simulink model "v09_threebit_mult"  (R2019b)
settings: Solver=FixedStepAuto  StartTime=0.0  StopTime=inf  FixedStep=1  MaxStep=1  RelTol=1e-3
libraries: simulink x6
settings Model: Creator=MARAT  LastModifiedBy=Marat
settings SFSimCC: CustomCodeUndefinedFunction=UseInterfaceOnly

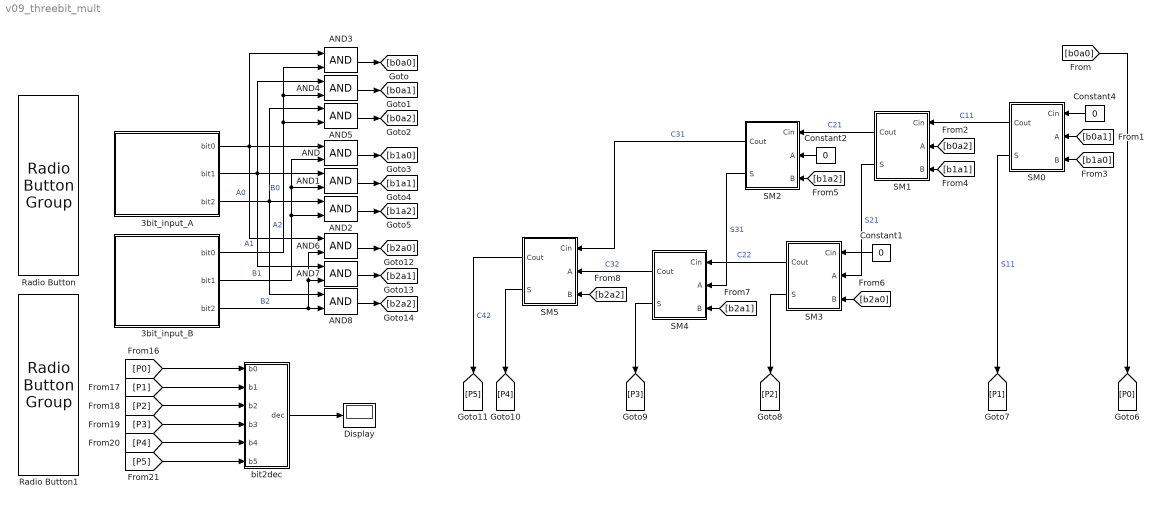
== system v09_threebit_mult ==
  3bit_input_A : Subsystem
      mask Display: image('images\sansA.png'); % Use "Edit Image" on toolstrip to change.
  3bit_input_B : Subsystem
      mask Display: image('images\sansB.png'); % Use "Edit Image" on toolstrip to change.
  AND{,1..8} (9 alike) : Logic  AllPortsSameDT=off  OutDataTypeStr=boolean
  Constant1 : Constant  Value=0  OutDataTypeStr=boolean
  Constant2 : Constant  Value=0  OutDataTypeStr=boolean
  Constant4 : Constant  Value=0  OutDataTypeStr=boolean
  Display : Display
  Radio Button : RadioButtonGroup  SelectedLabel=0
      settings: Values={{'0', '1', '2', '3', '4', '5', '6', '7'}, [0 1 2 3 4 5 6 7]}
  Radio Button1 : RadioButtonGroup  SelectedLabel=0
      settings: Values={{'0', '1', '2', '3', '4', '5', '6', '7'}, [0 1 2 3 4 5 6 7]}
  SM0 : Subsystem
  SM1 : Subsystem
  SM2 : Subsystem
  SM3 : Subsystem
  SM4 : Subsystem
  SM5 : Subsystem
  bit2dec : Subsystem
  wires:
  Constant4/1 -> SM0/1(Cin)
  [b0a0] -> [P0]
  3bit_input_A/1(bit0) -> AND6/1, AND/1, AND3/1  "A0"
  3bit_input_A/3(bit2) -> AND8/1, AND5/1, AND2/1  "A2"
  3bit_input_B/2(bit1) -> AND2/2, AND1/2, AND/2  "B1"
  [P0] -> bit2dec/1(b0)
  [P1] -> bit2dec/2(b1)
  [P2] -> bit2dec/3(b2)
  [P3] -> bit2dec/4(b3)
  [P4] -> bit2dec/5(b4)
  [P5] -> bit2dec/6(b5)
  bit2dec/1(dec) -> Display/1
  3bit_input_B/3(bit2) -> AND6/2, AND7/2, AND8/2  "B2"
  SM0/2(S) -> [P1]  "S11"
  SM1/1(Cout) -> SM2/1(Cin)  "C21"
  SM1/2(S) -> SM3/2(A)  "S21"
  SM3/2(S) -> [P2]
  SM3/1(Cout) -> SM4/1(Cin)  "C22"
  SM2/2(S) -> SM4/2(A)  "S31"
  SM4/2(S) -> [P3]
  3bit_input_A/2(bit1) -> AND7/1, AND4/1, AND1/1  "A1"
  3bit_input_B/1(bit0) -> AND3/2, AND4/2, AND5/2  "B0"
  AND3/1 -> [b0a0]
  AND4/1 -> [b0a1]
  AND5/1 -> [b0a2]
  AND2/1 -> [b1a2]
  AND1/1 -> [b1a1]
  AND/1 -> [b1a0]
  AND6/1 -> [b2a0]
  AND7/1 -> [b2a1]
  AND8/1 -> [b2a2]
  [b1a0] -> SM0/3(B)
  [b0a1] -> SM0/2(A)
  [b1a1] -> SM1/3(B)
  [b0a2] -> SM1/2(A)
  [b1a2] -> SM2/3(B)
  [b2a1] -> SM4/3(B)
  [b2a0] -> SM3/3(B)
  SM0/1(Cout) -> SM1/1(Cin)  "C11"
  Constant2/1 -> SM2/2(A)
  SM2/1(Cout) -> SM5/1(Cin)  "C31"
  [b2a2] -> SM5/3(B)
  SM4/1(Cout) -> SM5/2(A)  "C32"
  SM5/2(S) -> [P4]
  SM5/1(Cout) -> [P5]  "C42"
  Constant1/1 -> SM3/1(Cin)

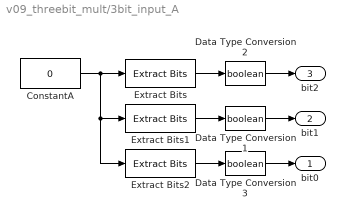
== system v09_threebit_mult/3bit_input_A ==
  ConstantA : Constant  Value=0  OutMin=0  OutMax=7  OutDataTypeStr=uint8
  Data Type Conversion1 : DataTypeConversion  OutDataTypeStr=boolean
  Data Type Conversion2 : DataTypeConversion  OutDataTypeStr=boolean
  Data Type Conversion3 : DataTypeConversion  OutDataTypeStr=boolean
  Extract Bits : simulink/Logic and Bit Operations/Extract Bits  bitsToExtract=Range of bits  numBits=8  bitIdxRange=2  outScalingMode=Treat bit field as an integer
      settings: SourceProductName=Simulink
  Extract Bits1 : simulink/Logic and Bit Operations/Extract Bits  bitsToExtract=Range of bits  numBits=8  bitIdxRange=1  outScalingMode=Treat bit field as an integer
      settings: SourceProductName=Simulink
  Extract Bits2 : simulink/Logic and Bit Operations/Extract Bits  bitsToExtract=Range of bits  numBits=8  bitIdxRange=0  outScalingMode=Treat bit field as an integer
      settings: SourceProductName=Simulink
  bit0 : Outport
  bit1 : Outport  Port=2
  bit2 : Outport  Port=3
  wires:
  ConstantA/1 -> Extract Bits2/1, Extract Bits1/1, Extract Bits/1
  Extract Bits/1 -> Data Type Conversion2/1
  Extract Bits1/1 -> Data Type Conversion1/1
  Extract Bits2/1 -> Data Type Conversion3/1
  Data Type Conversion2/1 -> bit2/1
  Data Type Conversion1/1 -> bit1/1
  Data Type Conversion3/1 -> bit0/1

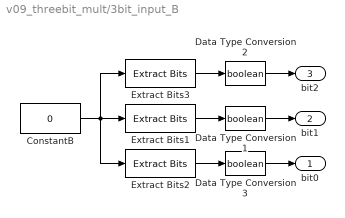
== system v09_threebit_mult/3bit_input_B ==
  ConstantB : Constant  Value=0  OutMin=0  OutMax=7  OutDataTypeStr=uint8
  Data Type Conversion1 : DataTypeConversion  OutDataTypeStr=boolean
  Data Type Conversion2 : DataTypeConversion  OutDataTypeStr=boolean
  Data Type Conversion3 : DataTypeConversion  OutDataTypeStr=boolean
  Extract Bits1 : simulink/Logic and Bit Operations/Extract Bits  bitsToExtract=Range of bits  numBits=8  bitIdxRange=1  outScalingMode=Treat bit field as an integer
      settings: SourceProductName=Simulink
  Extract Bits2 : simulink/Logic and Bit Operations/Extract Bits  bitsToExtract=Range of bits  numBits=8  bitIdxRange=0  outScalingMode=Treat bit field as an integer
      settings: SourceProductName=Simulink
  Extract Bits3 : simulink/Logic and Bit Operations/Extract Bits  bitsToExtract=Range of bits  numBits=8  bitIdxRange=2  outScalingMode=Treat bit field as an integer
      settings: SourceProductName=Simulink
  bit0 : Outport
  bit1 : Outport  Port=2
  bit2 : Outport  Port=3
  wires:
  Data Type Conversion3/1 -> bit0/1
  Data Type Conversion1/1 -> bit1/1
  Extract Bits2/1 -> Data Type Conversion3/1
  Extract Bits1/1 -> Data Type Conversion1/1
  ConstantB/1 -> Extract Bits3/1, Extract Bits1/1, Extract Bits2/1
  Extract Bits3/1 -> Data Type Conversion2/1
  Data Type Conversion2/1 -> bit2/1

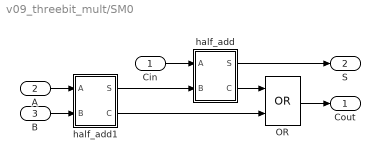
== system v09_threebit_mult/SM0 ==
  Cin : Inport
  A : Inport  Port=2
  B : Inport  Port=3
  OR : Logic  Operator=OR  AllPortsSameDT=off  OutDataTypeStr=boolean
  half_add : Subsystem
  half_add1 : Subsystem
  Cout : Outport
  S : Outport  Port=2
  wires:
  half_add/1(S) -> S/1
  A/1 -> half_add1/1(A)
  half_add/2(C) -> OR/1
  half_add1/1(S) -> half_add/2(B)
  B/1 -> half_add1/2(B)
  Cin/1 -> half_add/1(A)
  OR/1 -> Cout/1
  half_add1/2(C) -> OR/2

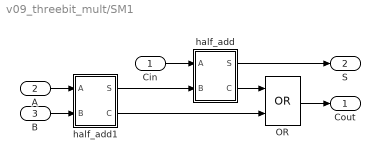
== system v09_threebit_mult/SM1 ==
  Cin : Inport
  A : Inport  Port=2
  B : Inport  Port=3
  OR : Logic  Operator=OR  AllPortsSameDT=off  OutDataTypeStr=boolean
  half_add : Subsystem
  half_add1 : Subsystem
  Cout : Outport
  S : Outport  Port=2
  wires:
  half_add1/2(C) -> OR/2
  OR/1 -> Cout/1
  Cin/1 -> half_add/1(A)
  B/1 -> half_add1/2(B)
  half_add1/1(S) -> half_add/2(B)
  half_add/2(C) -> OR/1
  A/1 -> half_add1/1(A)
  half_add/1(S) -> S/1

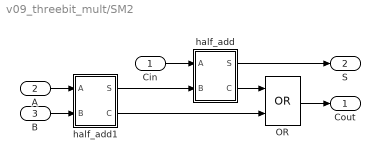
== system v09_threebit_mult/SM2 ==
  Cin : Inport
  A : Inport  Port=2
  B : Inport  Port=3
  OR : Logic  Operator=OR  AllPortsSameDT=off  OutDataTypeStr=boolean
  half_add : Subsystem
  half_add1 : Subsystem
  Cout : Outport
  S : Outport  Port=2
  wires:
  half_add/1(S) -> S/1
  A/1 -> half_add1/1(A)
  half_add/2(C) -> OR/1
  half_add1/1(S) -> half_add/2(B)
  B/1 -> half_add1/2(B)
  Cin/1 -> half_add/1(A)
  OR/1 -> Cout/1
  half_add1/2(C) -> OR/2

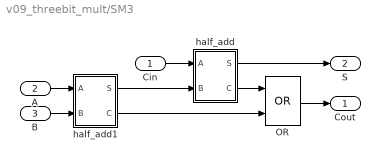
== system v09_threebit_mult/SM3 ==
  Cin : Inport
  A : Inport  Port=2
  B : Inport  Port=3
  OR : Logic  Operator=OR  AllPortsSameDT=off  OutDataTypeStr=boolean
  half_add : Subsystem
  half_add1 : Subsystem
  Cout : Outport
  S : Outport  Port=2
  wires:
  half_add1/2(C) -> OR/2
  OR/1 -> Cout/1
  Cin/1 -> half_add/1(A)
  B/1 -> half_add1/2(B)
  half_add1/1(S) -> half_add/2(B)
  half_add/2(C) -> OR/1
  A/1 -> half_add1/1(A)
  half_add/1(S) -> S/1

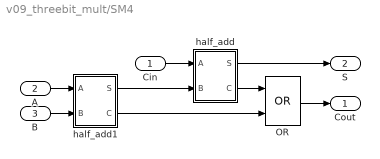
== system v09_threebit_mult/SM4 ==
  Cin : Inport
  A : Inport  Port=2
  B : Inport  Port=3
  OR : Logic  Operator=OR  AllPortsSameDT=off  OutDataTypeStr=boolean
  half_add : Subsystem
  half_add1 : Subsystem
  Cout : Outport
  S : Outport  Port=2
  wires:
  half_add/1(S) -> S/1
  A/1 -> half_add1/1(A)
  half_add/2(C) -> OR/1
  half_add1/1(S) -> half_add/2(B)
  B/1 -> half_add1/2(B)
  Cin/1 -> half_add/1(A)
  OR/1 -> Cout/1
  half_add1/2(C) -> OR/2

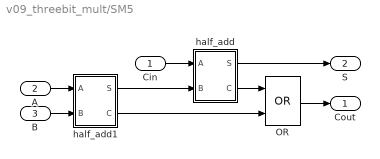
== system v09_threebit_mult/SM5 ==
  Cin : Inport
  A : Inport  Port=2
  B : Inport  Port=3
  OR : Logic  Operator=OR  AllPortsSameDT=off  OutDataTypeStr=boolean
  half_add : Subsystem
  half_add1 : Subsystem
  Cout : Outport
  S : Outport  Port=2
  wires:
  half_add1/2(C) -> OR/2
  OR/1 -> Cout/1
  Cin/1 -> half_add/1(A)
  B/1 -> half_add1/2(B)
  half_add1/1(S) -> half_add/2(B)
  half_add/2(C) -> OR/1
  A/1 -> half_add1/1(A)
  half_add/1(S) -> S/1

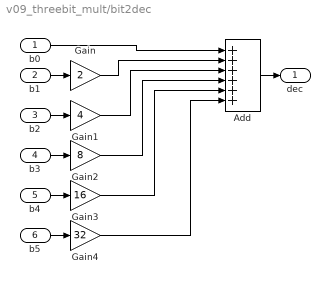
== system v09_threebit_mult/bit2dec ==
  b0 : Inport
  b1 : Inport  Port=2
  b2 : Inport  Port=3
  b3 : Inport  Port=4
  b4 : Inport  Port=5
  b5 : Inport  Port=6
  Add : Sum  Inputs=++++++
  Gain : Gain  Gain=2
  Gain1 : Gain  Gain=4
  Gain2 : Gain  Gain=8
  Gain3 : Gain  Gain=16
  Gain4 : Gain  Gain=32
  dec : Outport
  wires:
  b1/1 -> Gain/1
  b3/1 -> Gain2/1
  b2/1 -> Gain1/1
  b0/1 -> Add/1
  Add/1 -> dec/1
  Gain/1 -> Add/2
  Gain1/1 -> Add/3
  Gain2/1 -> Add/4
  b4/1 -> Gain3/1
  Gain3/1 -> Add/5
  Gain4/1 -> Add/6
  b5/1 -> Gain4/1

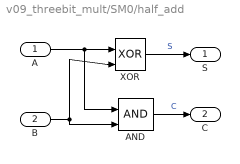
== system v09_threebit_mult/SM0/half_add ==
  A : Inport
  B : Inport  Port=2
  AND : Logic  IconShape=distinctive  AllPortsSameDT=off  OutDataTypeStr=boolean
  XOR : Logic  Operator=XOR  IconShape=distinctive  AllPortsSameDT=off  OutDataTypeStr=boolean
  S : Outport
  C : Outport  Port=2
  wires:
  XOR/1 -> S/1  "S"
  B/1 -> AND/2, XOR/2
  A/1 -> AND/1, XOR/1
  AND/1 -> C/1  "C"

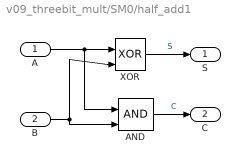
== system v09_threebit_mult/SM0/half_add1 ==
  A : Inport
  B : Inport  Port=2
  AND : Logic  IconShape=distinctive  AllPortsSameDT=off  OutDataTypeStr=boolean
  XOR : Logic  Operator=XOR  IconShape=distinctive  AllPortsSameDT=off  OutDataTypeStr=boolean
  S : Outport
  C : Outport  Port=2
  wires:
  AND/1 -> C/1  "C"
  A/1 -> XOR/1, AND/1
  B/1 -> XOR/2, AND/2
  XOR/1 -> S/1  "S"

== system v09_threebit_mult/SM1/half_add ==
  A : Inport
  B : Inport  Port=2
  AND : Logic  IconShape=distinctive  AllPortsSameDT=off  OutDataTypeStr=boolean
  XOR : Logic  Operator=XOR  IconShape=distinctive  AllPortsSameDT=off  OutDataTypeStr=boolean
  S : Outport
  C : Outport  Port=2
  wires:
  AND/1 -> C/1  "C"
  A/1 -> XOR/1, AND/1
  B/1 -> XOR/2, AND/2
  XOR/1 -> S/1  "S"

== system v09_threebit_mult/SM1/half_add1 ==
  A : Inport
  B : Inport  Port=2
  AND : Logic  IconShape=distinctive  AllPortsSameDT=off  OutDataTypeStr=boolean
  XOR : Logic  Operator=XOR  IconShape=distinctive  AllPortsSameDT=off  OutDataTypeStr=boolean
  S : Outport
  C : Outport  Port=2
  wires:
  XOR/1 -> S/1  "S"
  B/1 -> AND/2, XOR/2
  A/1 -> AND/1, XOR/1
  AND/1 -> C/1  "C"

== system v09_threebit_mult/SM2/half_add ==
  A : Inport
  B : Inport  Port=2
  AND : Logic  IconShape=distinctive  AllPortsSameDT=off  OutDataTypeStr=boolean
  XOR : Logic  Operator=XOR  IconShape=distinctive  AllPortsSameDT=off  OutDataTypeStr=boolean
  S : Outport
  C : Outport  Port=2
  wires:
  XOR/1 -> S/1  "S"
  B/1 -> AND/2, XOR/2
  A/1 -> AND/1, XOR/1
  AND/1 -> C/1  "C"

== system v09_threebit_mult/SM2/half_add1 ==
  A : Inport
  B : Inport  Port=2
  AND : Logic  IconShape=distinctive  AllPortsSameDT=off  OutDataTypeStr=boolean
  XOR : Logic  Operator=XOR  IconShape=distinctive  AllPortsSameDT=off  OutDataTypeStr=boolean
  S : Outport
  C : Outport  Port=2
  wires:
  AND/1 -> C/1  "C"
  A/1 -> XOR/1, AND/1
  B/1 -> XOR/2, AND/2
  XOR/1 -> S/1  "S"

== system v09_threebit_mult/SM3/half_add ==
  A : Inport
  B : Inport  Port=2
  AND : Logic  IconShape=distinctive  AllPortsSameDT=off  OutDataTypeStr=boolean
  XOR : Logic  Operator=XOR  IconShape=distinctive  AllPortsSameDT=off  OutDataTypeStr=boolean
  S : Outport
  C : Outport  Port=2
  wires:
  AND/1 -> C/1  "C"
  A/1 -> XOR/1, AND/1
  B/1 -> XOR/2, AND/2
  XOR/1 -> S/1  "S"

== system v09_threebit_mult/SM3/half_add1 ==
  A : Inport
  B : Inport  Port=2
  AND : Logic  IconShape=distinctive  AllPortsSameDT=off  OutDataTypeStr=boolean
  XOR : Logic  Operator=XOR  IconShape=distinctive  AllPortsSameDT=off  OutDataTypeStr=boolean
  S : Outport
  C : Outport  Port=2
  wires:
  XOR/1 -> S/1  "S"
  B/1 -> AND/2, XOR/2
  A/1 -> AND/1, XOR/1
  AND/1 -> C/1  "C"

== system v09_threebit_mult/SM4/half_add ==
  A : Inport
  B : Inport  Port=2
  AND : Logic  IconShape=distinctive  AllPortsSameDT=off  OutDataTypeStr=boolean
  XOR : Logic  Operator=XOR  IconShape=distinctive  AllPortsSameDT=off  OutDataTypeStr=boolean
  S : Outport
  C : Outport  Port=2
  wires:
  XOR/1 -> S/1  "S"
  B/1 -> AND/2, XOR/2
  A/1 -> AND/1, XOR/1
  AND/1 -> C/1  "C"

== system v09_threebit_mult/SM4/half_add1 ==
  A : Inport
  B : Inport  Port=2
  AND : Logic  IconShape=distinctive  AllPortsSameDT=off  OutDataTypeStr=boolean
  XOR : Logic  Operator=XOR  IconShape=distinctive  AllPortsSameDT=off  OutDataTypeStr=boolean
  S : Outport
  C : Outport  Port=2
  wires:
  AND/1 -> C/1  "C"
  A/1 -> XOR/1, AND/1
  B/1 -> XOR/2, AND/2
  XOR/1 -> S/1  "S"

== system v09_threebit_mult/SM5/half_add ==
  A : Inport
  B : Inport  Port=2
  AND : Logic  IconShape=distinctive  AllPortsSameDT=off  OutDataTypeStr=boolean
  XOR : Logic  Operator=XOR  IconShape=distinctive  AllPortsSameDT=off  OutDataTypeStr=boolean
  S : Outport
  C : Outport  Port=2
  wires:
  AND/1 -> C/1  "C"
  A/1 -> XOR/1, AND/1
  B/1 -> XOR/2, AND/2
  XOR/1 -> S/1  "S"

== system v09_threebit_mult/SM5/half_add1 ==
  A : Inport
  B : Inport  Port=2
  AND : Logic  IconShape=distinctive  AllPortsSameDT=off  OutDataTypeStr=boolean
  XOR : Logic  Operator=XOR  IconShape=distinctive  AllPortsSameDT=off  OutDataTypeStr=boolean
  S : Outport
  C : Outport  Port=2
  wires:
  XOR/1 -> S/1  "S"
  B/1 -> AND/2, XOR/2
  A/1 -> AND/1, XOR/1
  AND/1 -> C/1  "C"
